simulink model "task_simulation"  (R2025b)
settings: Solver=FixedStepAuto  StartTime=0.0  StopTime=20  FixedStep=Ts * 0.1  RelTol=1e-3
InitFcn:
  | % modelling
  | % design_cascade_control
undefined symbols (not defined in the file): CTRL, I_max_val, J_1_val, J_2_val, k_E_val, k_M_val, k_t_val, L_val, R_val, U_max_val
libraries: slpidlib x7, embmathops x2, simulink_extras x2, simulink x2
settings Model: Creator=10120  LastModifiedBy=10120
settings SolverCC: ZeroCrossAlgorithm=Adaptive
settings DebuggingCC: IgnoredZcDiagnostic=none

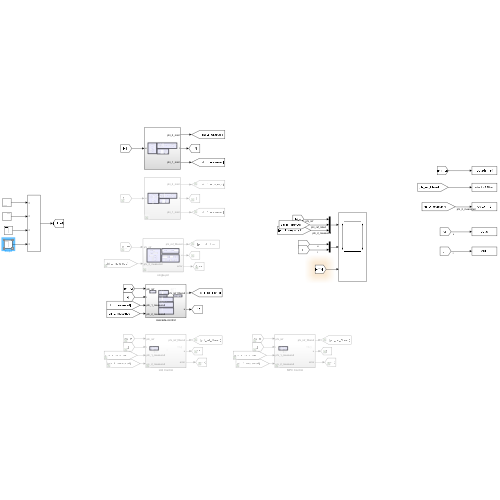
[thumbnail: Simulink's stored preview of the top-level diagram]
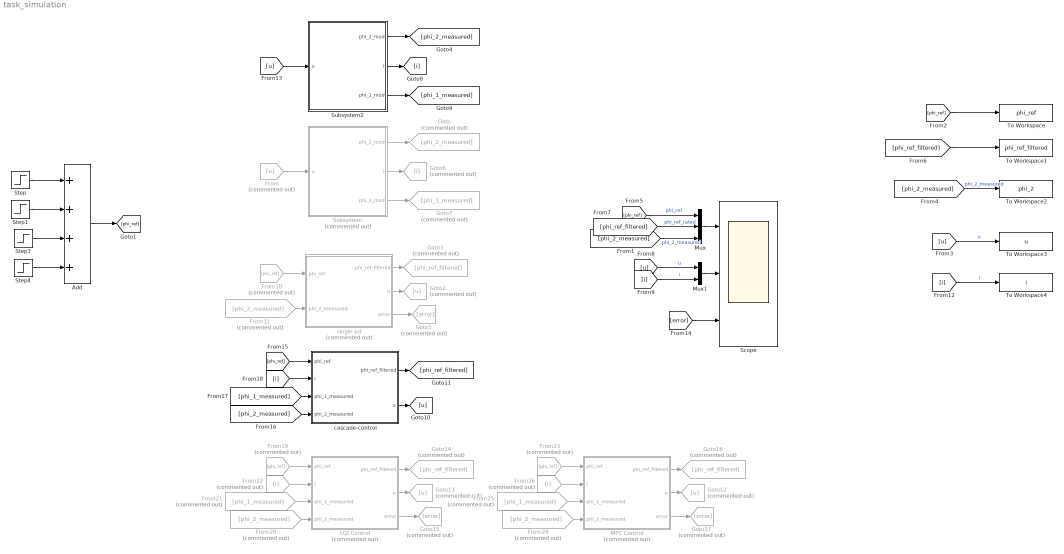
== system task_simulation ==
  Add : Sum  Inputs=++++
  From : From  Commented=on  GotoTag=u
  From10 : From  Commented=on  GotoTag=phi_ref
  From11 : From  Commented=on  GotoTag=phi_2_measured
  From19 : From  Commented=on  GotoTag=phi_ref
  From20 : From  Commented=on  GotoTag=phi_2_measured
  From21 : From  Commented=on  GotoTag=phi_1_measured
  From22 : From  Commented=on  GotoTag=i
  From23 : From  Commented=on  GotoTag=phi_ref
  From24 : From  Commented=on  GotoTag=phi_2_measured
  From25 : From  Commented=on  GotoTag=phi_1_measured
  From26 : From  Commented=on  GotoTag=i
  Goto : Goto  Commented=on  GotoTag=phi_2_measured
  Goto12 : Goto  Commented=on  GotoTag=u
  Goto13 : Goto  Commented=on  GotoTag=u
  Goto14 : Goto  Commented=on  GotoTag=phi_ref_filtered
  Goto15 : Goto  Commented=on  GotoTag=error
  Goto16 : Goto  Commented=on  GotoTag=phi_ref_filtered
  Goto17 : Goto  Commented=on  GotoTag=error
  Goto2 : Goto  Commented=on  GotoTag=u
  Goto3 : Goto  Commented=on  GotoTag=phi_ref_filtered
  Goto5 : Goto  Commented=on  GotoTag=error
  Goto6 : Goto  Commented=on  GotoTag=i
  Goto7 : Goto  Commented=on  GotoTag=phi_1_measured
  LQI Control : Subsystem  Commented=on
  MPC Control : Subsystem  Commented=on
  Mux : Mux  Inputs=3
  Mux1 : Mux  Inputs=2
  Scope : Scope  NumInputPorts=3
      settings: ActiveDisplayYMinimum=-0.74999999999999978  ActiveDisplayYMaximum=6.75
  Step : Step  Time=0.1  After=2  SampleTime=0
  Step1 : Step  Time=5  After=2  SampleTime=0
  Step3 : Step  Time=10  After=-2  SampleTime=0
  Step4 : Step  Time=15  After=-2  SampleTime=0
  Subsystem : Subsystem  Commented=on
  Subsystem2 : Subsystem
  To Workspace : ToWorkspace  VariableName=phi_ref  SaveFormat=Structure With Time  SampleTime=-1
  To Workspace1 : ToWorkspace  VariableName=phi_ref_filtered  SaveFormat=Structure With Time  SampleTime=-1
  To Workspace2 : ToWorkspace  VariableName=phi_2  SaveFormat=Structure With Time  SampleTime=-1
  To Workspace3 : ToWorkspace  VariableName=u  SaveFormat=Structure With Time  SampleTime=-1
  To Workspace4 : ToWorkspace  VariableName=i  SaveFormat=Structure With Time  SampleTime=-1
  cascade-control : Subsystem
  single-pd : Subsystem  Commented=on
  wires:
  From/1 -> Subsystem/1(u)
  Subsystem/1(phi_2_mod) -> Goto/1
  Mux/1 -> Scope/1
  [phi_ref] -> Mux/1  "phi_ref"
  [phi_ref_filtered] -> Mux/2  "phi_ref_rated"
  [phi_2_measured] -> Mux/3  "phi_2_measured"
  Subsystem/2(i) -> Goto6/1
  From10/1 -> single-pd/1(phi_ref)
  From11/1 -> single-pd/2(phi_2_measured)
  single-pd/2(u) -> Goto2/1
  single-pd/1(phi_ref_filtered) -> Goto3/1
  Mux1/1 -> Scope/2
  [u] -> Mux1/1  "u"
  [i] -> Mux1/2  "i"
  [phi_ref] -> To Workspace/1
  [phi_ref_filtered] -> To Workspace1/1
  [phi_2_measured] -> To Workspace2/1  "phi_2_measured"
  [u] -> To Workspace3/1  "u"
  [i] -> To Workspace4/1  "i"
  single-pd/3(error) -> Goto5/1
  [error] -> Scope/3
  Subsystem/3(phi_1_mod) -> Goto7/1
  Subsystem2/3(phi_1_mod) -> [phi_1_measured]
  Subsystem2/2(i) -> [i]
  Subsystem2/1(phi_2_mod) -> [phi_2_measured]
  [u] -> Subsystem2/1(u)
  [phi_ref] -> cascade-control/1(phi_ref)
  cascade-control/1(phi_ref_filtered) -> [phi_ref_filtered]
  [phi_2_measured] -> cascade-control/4(phi_2_measured)
  cascade-control/2(u) -> [u]
  [phi_1_measured] -> cascade-control/3(phi_1_measured)
  [i] -> cascade-control/2(i)
  From22/1 -> LQI Control/2(i)
  LQI Control/1(phi_ref_filtered) -> Goto14/1
  From21/1 -> LQI Control/3(phi_1_measured)
  LQI Control/2(u) -> Goto13/1
  From19/1 -> LQI Control/1(phi_ref)
  From20/1 -> LQI Control/4(phi_2_measured)
  LQI Control/3(error) -> Goto15/1
  From25/1 -> MPC Control/3(phi_1_measured)
  From23/1 -> MPC Control/1(phi_ref)
  MPC Control/1(phi_ref_filtered) -> Goto16/1
  From24/1 -> MPC Control/4(phi_2_measured)
  MPC Control/2(u) -> Goto12/1
  From26/1 -> MPC Control/2(i)
  MPC Control/3(error) -> Goto17/1
  Step/1 -> Add/1
  Step1/1 -> Add/2
  Step3/1 -> Add/3
  Step4/1 -> Add/4
  Add/1 -> [phi_ref]

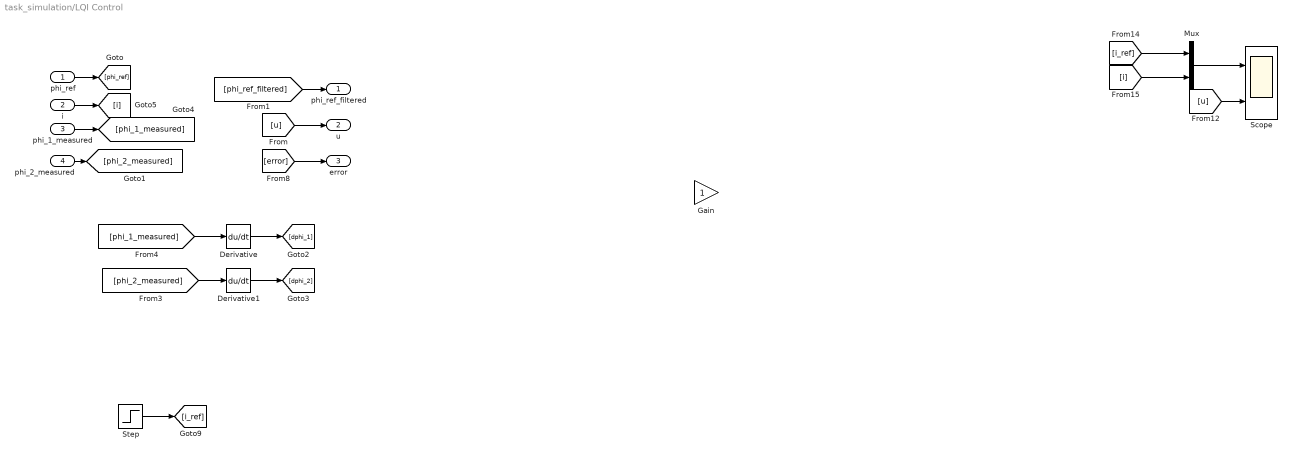
== system task_simulation/LQI Control ==
  phi_ref : Inport
  i : Inport  Port=2
  phi_1_measured : Inport  Port=3
  phi_2_measured : Inport  Port=4
  Derivative : Derivative
  Derivative1 : Derivative
  Gain : Gain
  Mux : Mux  Inputs=2
  Scope : Scope  NumInputPorts=2
      settings: ActiveDisplayYMinimum=-0.12500000000858569  ActiveDisplayYMaximum=1.1250000000772715
  Step : Step  SampleTime=0
  phi_ref_filtered : Outport
  u : Outport  Port=2
  error : Outport  Port=3
  wires:
  phi_ref/1 -> [phi_ref]
  phi_2_measured/1 -> [phi_2_measured]
  [phi_ref_filtered] -> phi_ref_filtered/1
  [u] -> u/1
  [error] -> error/1
  [phi_1_measured] -> Derivative/1
  Derivative/1 -> [dphi_1]
  [phi_2_measured] -> Derivative1/1
  Derivative1/1 -> [dphi_2]
  phi_1_measured/1 -> [phi_1_measured]
  i/1 -> [i]
  [i_ref] -> Mux/1
  [i] -> Mux/2
  Mux/1 -> Scope/1
  [u] -> Scope/2
  Step/1 -> [i_ref]

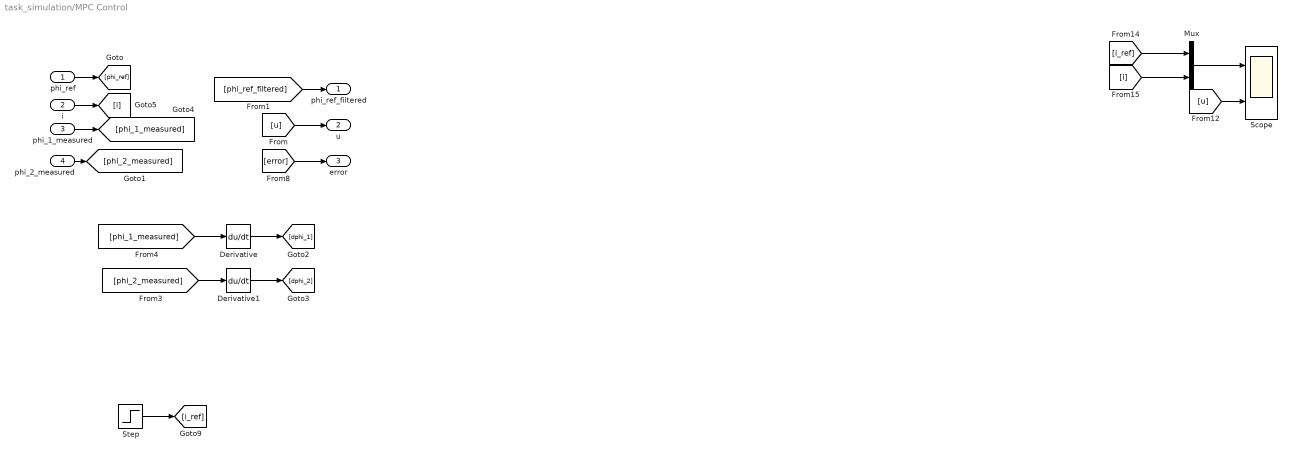
== system task_simulation/MPC Control ==
  phi_ref : Inport
  i : Inport  Port=2
  phi_1_measured : Inport  Port=3
  phi_2_measured : Inport  Port=4
  Derivative : Derivative
  Derivative1 : Derivative
  Mux : Mux  Inputs=2
  Scope : Scope  NumInputPorts=2
      settings: ActiveDisplayYMinimum=-0.12500000000858569  ActiveDisplayYMaximum=1.1250000000772715
  Step : Step  SampleTime=0
  phi_ref_filtered : Outport
  u : Outport  Port=2
  error : Outport  Port=3
  wires:
  phi_ref/1 -> [phi_ref]
  phi_2_measured/1 -> [phi_2_measured]
  [phi_ref_filtered] -> phi_ref_filtered/1
  [u] -> u/1
  [error] -> error/1
  [phi_1_measured] -> Derivative/1
  Derivative/1 -> [dphi_1]
  [phi_2_measured] -> Derivative1/1
  Derivative1/1 -> [dphi_2]
  phi_1_measured/1 -> [phi_1_measured]
  i/1 -> [i]
  [i_ref] -> Mux/1
  [i] -> Mux/2
  Mux/1 -> Scope/1
  [u] -> Scope/2
  Step/1 -> [i_ref]

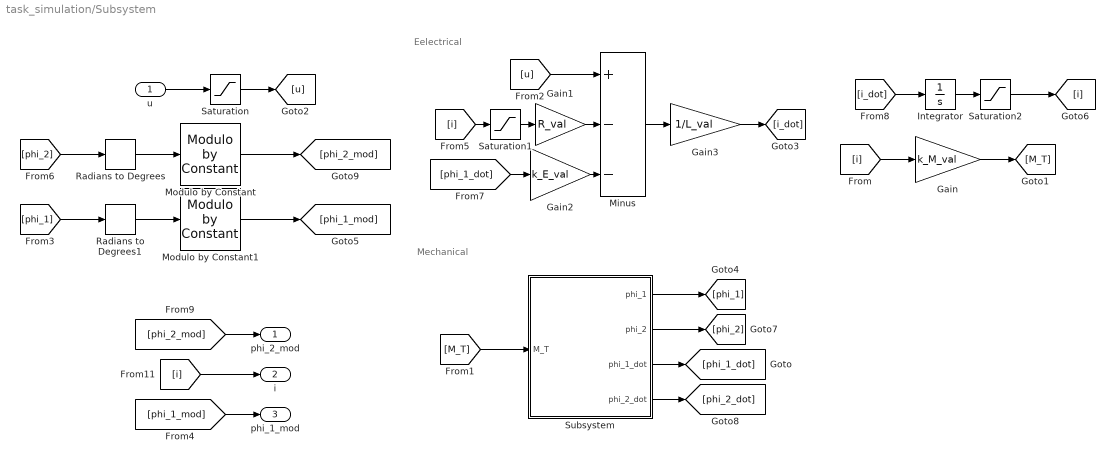
== system task_simulation/Subsystem ==
  note: Mechanical
  note: Eelectrical
  u : Inport
  Gain : Gain  Gain=k_M_val
  Gain1 : Gain  Gain=R_val
  Gain2 : Gain  Gain=k_E_val
  Gain3 : Gain  Gain=1/L_val
  Integrator : Integrator
  Minus : Sum  Inputs=+--
  Modulo by Constant : embmathops/Modulo by Constant  Denominator=360  SimulateUsing=Code generation
      settings: LibrarySourceBlock=embeddedMathLib/Modulo by Constant
  Modulo by Constant1 : embmathops/Modulo by Constant  Denominator=360  SimulateUsing=Code generation
      settings: LibrarySourceBlock=embeddedMathLib/Modulo by Constant
  Radians to Degrees : simulink_extras/Transformations/Radians to Degrees
  Radians to Degrees1 : simulink_extras/Transformations/Radians to Degrees
  Saturation : Saturate  UpperLimit=U_max_val  LowerLimit=-U_max_val
  Saturation1 : Saturate  UpperLimit=I_max_val  LowerLimit=-I_max_val
  Saturation2 : Saturate  UpperLimit=I_max_val  LowerLimit=-I_max_val
  Subsystem : Subsystem
  phi_2_mod : Outport
  i : Outport  Port=2
  phi_1_mod : Outport  Port=3
  wires:
  [i] -> Gain/1
  Gain/1 -> [M_T]
  [M_T] -> Subsystem/1(M_T)
  u/1 -> Saturation/1
  Gain3/1 -> [i_dot]
  [u] -> Minus/1
  Gain1/1 -> Minus/2
  [i] -> Saturation1/1
  Subsystem/1(phi_1) -> [phi_1]
  Gain2/1 -> Minus/3
  [phi_1_dot] -> Gain2/1
  Minus/1 -> Gain3/1
  [i_dot] -> Integrator/1
  Integrator/1 -> Saturation2/1
  Subsystem/3(phi_1_dot) -> [phi_1_dot]
  [phi_2_mod] -> phi_2_mod/1
  Subsystem/2(phi_2) -> [phi_2]
  Subsystem/4(phi_2_dot) -> [phi_2_dot]
  [phi_2] -> Radians to Degrees/1
  Saturation/1 -> [u]
  Saturation1/1 -> Gain1/1
  Saturation2/1 -> [i]
  [i] -> i/1
  Radians to Degrees/1 -> Modulo by Constant/1
  Modulo by Constant/1 -> [phi_2_mod]
  Radians to Degrees1/1 -> Modulo by Constant1/1
  [phi_1] -> Radians to Degrees1/1
  Modulo by Constant1/1 -> [phi_1_mod]
  [phi_1_mod] -> phi_1_mod/1

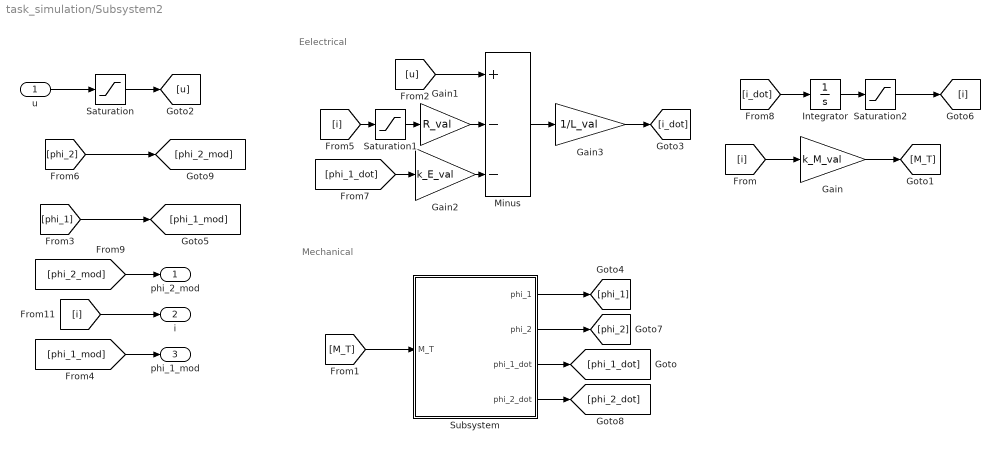
== system task_simulation/Subsystem2 ==
  note: Mechanical
  note: Eelectrical
  u : Inport
  Gain : Gain  Gain=k_M_val
  Gain1 : Gain  Gain=R_val
  Gain2 : Gain  Gain=k_E_val
  Gain3 : Gain  Gain=1/L_val
  Integrator : Integrator
  Minus : Sum  Inputs=+--
  Saturation : Saturate  UpperLimit=U_max_val  LowerLimit=-U_max_val
  Saturation1 : Saturate  UpperLimit=I_max_val  LowerLimit=-I_max_val
  Saturation2 : Saturate  UpperLimit=I_max_val  LowerLimit=-I_max_val
  Subsystem : Subsystem
  phi_2_mod : Outport
  i : Outport  Port=2
  phi_1_mod : Outport  Port=3
  wires:
  [i] -> Gain/1
  Gain/1 -> [M_T]
  [M_T] -> Subsystem/1(M_T)
  u/1 -> Saturation/1
  Gain3/1 -> [i_dot]
  [u] -> Minus/1
  Gain1/1 -> Minus/2
  [i] -> Saturation1/1
  Subsystem/1(phi_1) -> [phi_1]
  Gain2/1 -> Minus/3
  [phi_1_dot] -> Gain2/1
  Minus/1 -> Gain3/1
  [i_dot] -> Integrator/1
  Integrator/1 -> Saturation2/1
  Subsystem/3(phi_1_dot) -> [phi_1_dot]
  [phi_2_mod] -> phi_2_mod/1
  Subsystem/2(phi_2) -> [phi_2]
  Subsystem/4(phi_2_dot) -> [phi_2_dot]
  Saturation/1 -> [u]
  Saturation1/1 -> Gain1/1
  Saturation2/1 -> [i]
  [i] -> i/1
  [phi_2] -> [phi_2_mod]
  [phi_1] -> [phi_1_mod]
  [phi_1_mod] -> phi_1_mod/1

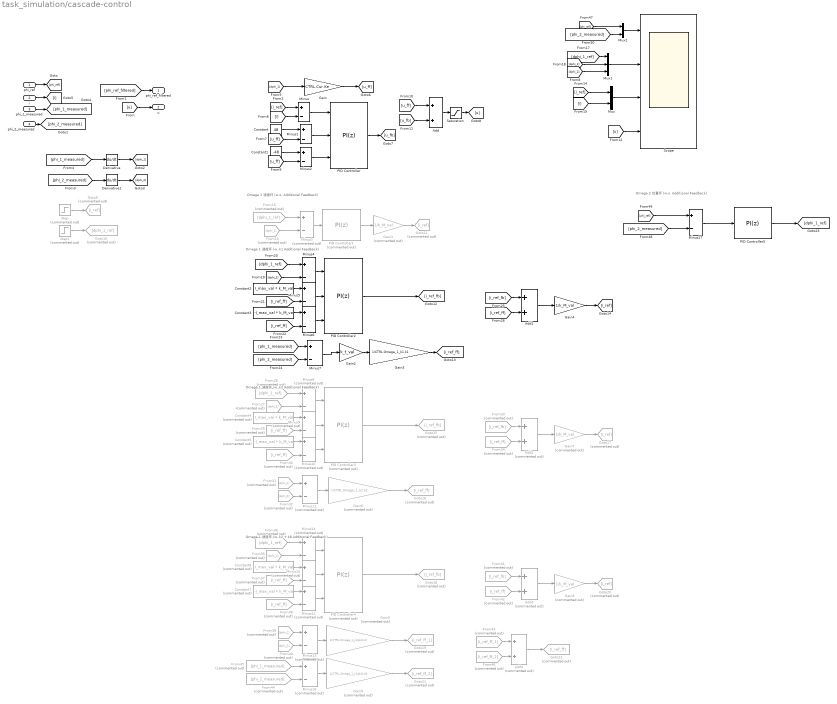
== system task_simulation/cascade-control ==
  note: Omega 1 速度环 (w. k1 Additional Feedback)
  note: Omega 1 速度环 (w.o. Additional Feedback)
  note: Omega 1 速度环 (w. k2 Additional Feedback)
  note: Omega 1 速度环 (w. k2 + k8 Additional Feedback)
  note: Omega 2 位置环 (w.o. Additional Feedback)
  phi_ref : Inport
  i : Inport  Port=2
  phi_1_measured : Inport  Port=3
  phi_2_measured : Inport  Port=4
  Add : Sum
  Add1 : Sum
  Add2 : Sum  Commented=on
  Add3 : Sum  Commented=on
  Add4 : Sum  Commented=on
  Constant : Constant  Value=48
  Constant1 : Constant  Value=-48
  Constant2 : Constant  Value=I_max_val * k_M_val
  Constant3 : Constant  Value=-I_max_val * k_M_val
  Constant4 : Constant  Commented=on  Value=I_max_val * k_M_val
  Constant5 : Constant  Commented=on  Value=-I_max_val * k_M_val
  Constant6 : Constant  Commented=on  Value=I_max_val * k_M_val
  Constant7 : Constant  Commented=on  Value=-I_max_val * k_M_val
  Derivative : Derivative
  Derivative1 : Derivative
  From{13,27,31,35,39} (5 alike) : From  Commented=on  GotoTag=dphi_1
  From16 : From  Commented=on  GotoTag=dphi_1_ref
  From28 : From  Commented=on  GotoTag=dphi_1_ref
  From{29..30,34,37..38,42} (6 alike) : From  Commented=on  GotoTag=i_ref_ff
  From32 : From  Commented=on  GotoTag=dphi_2
  From33 : From  Commented=on  GotoTag=i_ref_fb
  From36 : From  Commented=on  GotoTag=dphi_1_ref
  From40 : From  Commented=on  GotoTag=dphi_2
  From41 : From  Commented=on  GotoTag=i_ref_fb
  From43 : From  Commented=on  GotoTag=i_ref_ff_1
  From44 : From  Commented=on  GotoTag=phi_2_measured
  From45 : From  Commented=on  GotoTag=phi_1_measured
  From46 : From  Commented=on  GotoTag=i_ref_ff_2
  Gain : Gain  Gain=CTRL.Cur.Ke
  Gain1 : Gain  Commented=on  Gain=1/k_M_val
  Gain2 : Gain  Gain=k_t_val
  Gain3 : Gain  Gain=1/CTRL.Omega_1_k1.k1
  Gain4 : Gain  Gain=1/k_M_val
  Gain5 : Gain  Commented=on  Gain=1/CTRL.Omega_1_k2pk8.k2
  Gain6 : Gain  Commented=on  Gain=1/CTRL.Omega_1_k2.k2
  Gain7 : Gain  Commented=on  Gain=1/k_M_val
  Gain8 : Gain  Commented=on  Gain=1/k_M_val
  Gain9 : Gain  Commented=on  Gain=1/CTRL.Omega_1_k2pk8.k8
  Goto10 : Goto  Commented=on  GotoTag=dphi_1_ref
  Goto{9,11,17,20} (4 alike) : Goto  Commented=on  GotoTag=i_ref
  Goto15 : Goto  Commented=on  GotoTag=i_ref_fb
  Goto16 : Goto  Commented=on  GotoTag=i_ref_ff
  Goto18 : Goto  Commented=on  GotoTag=i_ref_fb
  Goto19 : Goto  Commented=on  GotoTag=i_ref_ff_1
  Goto21 : Goto  Commented=on  GotoTag=i_ref_ff_2
  Goto22 : Goto  Commented=on  GotoTag=i_ref_ff
  Minus{,1..2,4..7,17} (8 alike) : Sum  Inputs=+-
  Minus{3,8..16} (10 alike) : Sum  Commented=on  Inputs=+-
  Mux : Mux  Inputs=2
  Mux1 : Mux  Inputs=3
  Mux2 : Mux  Inputs=2
  PID Controller : slpidlib/PID Controller  Controller=PI  Form=Parallel  TimeDomain=Discrete-time  UseExternalTs=off  SampleTime=-1  IntegratorMethod=Forward Euler  FilterMethod=Forward Euler  ControllerParametersSource=internal  P=CTRL.Cur.Kp  I=CTRL.Cur.Ki  UseKiTs=off  D=0  UseExternalDerivativeSource=off  N=100  UseFilter=on  TunerSelectOption=Transfer Function Based (PID Tuner App)  InitialConditionSource=internal  InitialConditionForIntegrator=0  InitialConditionForFilter=0  DifferentiatorICPrevScaledInput=0  ExternalReset=none  TrackingMode=off  Kt=1  LimitOutput=on  SatLimitsSource=external  UpperSaturationLimit=inf  LowerSaturationLimit=-inf  LinearizeAsGain=on  AntiWindupMode=clamping  Kb=1  LimitIntegrator=off  UpperIntegratorSaturationLimit=inf  LowerIntegratorSaturationLimit=-inf  POutMin=[]  POutMax=[]  IOutMin=[]  IOutMax=[]  DOutMin=[]  DOutMax=[]  NOutMin=[]  NOutMax=[]  SumOutMin=[]  SumOutMax=[]  SaturationOutMin=[]  SaturationOutMax=[]  PParamMin=[]  PParamMax=[]  IParamMin=[]  IParamMax=[]  DParamMin=[]  DParamMax=[]  NParamMin=[]  NParamMax=[]  KbParamMin=[]  KbParamMax=[]  KtParamMin=[]  KtParamMax=[]  KbOutMin=[]  KbOutMax=[]  KtOutMin=[]  KtOutMax=[]  IntegratorOutMin=[]  IntegratorOutMax=[]  FilterOutMin=[]  FilterOutMax=[]  SumI1OutMin=[]  SumI1OutMax=[]  SumI2OutMin=[]  SumI2OutMax=[]  SumI3OutMin=[]  SumI3OutMax=[]  SumI4OutMin=[]  SumI4OutMax=[]  SumDOutMin=[]  SumDOutMax=[]  DifferentiatorOutMin=[]  DifferentiatorOutMax=[]  FilterDiffOutCoefMin=[]  FilterDiffOutCoefMax=[]  ReciprocalOutMin=[]  ReciprocalOutMax=[]  SumDenOutMin=[]  SumDenOutMax=[]  SumNumOutMin=[]  SumNumOutMax=[]  DivideOutMin=[]  DivideOutMax=[]  UdiffTsProdOutMin=[]  UdiffTsProdOutMax=[]  NTsProdOutMin=[]  NTsProdOutMax=[]  UintegralTsProdOutMin=[]  UintegralTsProdOutMax=[]  UngainTsProdOutMin=[]  UngainTsProdOutMax=[]  ClampingZeroOutDataTypeStr=Inherit: Inherit via back propagation  ClampingZeroOutMin=[]  ClampingZeroOutMax=[]  FilterDenConstantOutDataTypeStr=Inherit: Inherit via back propagation  FilterDenConstantOutMin=[]  FilterDenConstantOutMax=[]  PCopyOutDataTypeStr=Inherit: Inherit via back propagation  PCopyOutMin=[]  PCopyOutMax=[]  NCopyOutDataTypeStr=Inherit: Inherit via back propagation  NCopyOutMin=[]  NCopyOutMax=[]  IntegratorContinuousStateAttributes=''  IntegratorStateMustResolveToSignalObject=off  IntegratorRTWStateStorageClass=Auto  FilterContinuousStateAttributes=''  FilterStateMustResolveToSignalObject=off  FilterRTWStateStorageClass=Auto  ParallelPVariant=InternalParameters  IdealPVariant=Disabled  IVariant=InternalParameters  DVariant=Disabled  IntegratorVariant=Discrete  SatVariant=External  AWVariant=DiscClampingParallel  PCopyVariant=Disabled  TRVariant=Disabled  FdbkBlocksVariant=Forward  IdealPFdbkVariant=Disabled  SatFdbkVariant=Disabled  DerivativeFilterVariant=Disabled  NVariant=Disabled  NCopyVariant=Disabled_SignalSpec  FilterICVariant=Disabled  IntegratorICVariant=InternalICs  ExternalResetVariant=Disabled  TRSumVariant=Passthrough  SumFdbkVariant=Disabled  SumVariant=Sum_PI  TsampFilterVariant=InternalTs  TsampNgainVariant=Passthrough  TsampIntegralVariant=Disabled_SignalSpec  ExternalSaturationOutDataTypeStr=Inherit: Same as second input  DerivativeSourceVariant=Disabled  PreIntVariant=InternalPreInt
  PID Controller1 : slpidlib/PID Controller  Commented=on  Controller=PI  Form=Parallel  TimeDomain=Discrete-time  UseExternalTs=off  SampleTime=-1  IntegratorMethod=Forward Euler  FilterMethod=Forward Euler  ControllerParametersSource=internal  P=CTRL.Omega_1.Kp  I=CTRL.Omega_1.Ki  UseKiTs=off  D=0  UseExternalDerivativeSource=off  N=100  UseFilter=on  TunerSelectOption=Transfer Function Based (PID Tuner App)  InitialConditionSource=internal  InitialConditionForIntegrator=0  InitialConditionForFilter=0  DifferentiatorICPrevScaledInput=0  ExternalReset=none  TrackingMode=off  Kt=1  LimitOutput=on  SatLimitsSource=internal  UpperSaturationLimit=I_max_val * k_M_val  LowerSaturationLimit=-I_max_val * k_M_val  LinearizeAsGain=on  AntiWindupMode=clamping  Kb=1  LimitIntegrator=off  UpperIntegratorSaturationLimit=inf  LowerIntegratorSaturationLimit=-inf  POutMin=[]  POutMax=[]  IOutMin=[]  IOutMax=[]  DOutMin=[]  DOutMax=[]  NOutMin=[]  NOutMax=[]  SumOutMin=[]  SumOutMax=[]  SaturationOutMin=[]  SaturationOutMax=[]  PParamMin=[]  PParamMax=[]  IParamMin=[]  IParamMax=[]  DParamMin=[]  DParamMax=[]  NParamMin=[]  NParamMax=[]  KbParamMin=[]  KbParamMax=[]  KtParamMin=[]  KtParamMax=[]  KbOutMin=[]  KbOutMax=[]  KtOutMin=[]  KtOutMax=[]  IntegratorOutMin=[]  IntegratorOutMax=[]  FilterOutMin=[]  FilterOutMax=[]  SumI1OutMin=[]  SumI1OutMax=[]  SumI2OutMin=[]  SumI2OutMax=[]  SumI3OutMin=[]  SumI3OutMax=[]  SumI4OutMin=[]  SumI4OutMax=[]  SumDOutMin=[]  SumDOutMax=[]  DifferentiatorOutMin=[]  DifferentiatorOutMax=[]  FilterDiffOutCoefMin=[]  FilterDiffOutCoefMax=[]  ReciprocalOutMin=[]  ReciprocalOutMax=[]  SumDenOutMin=[]  SumDenOutMax=[]  SumNumOutMin=[]  SumNumOutMax=[]  DivideOutMin=[]  DivideOutMax=[]  UdiffTsProdOutMin=[]  UdiffTsProdOutMax=[]  NTsProdOutMin=[]  NTsProdOutMax=[]  UintegralTsProdOutMin=[]  UintegralTsProdOutMax=[]  UngainTsProdOutMin=[]  UngainTsProdOutMax=[]  ClampingZeroOutDataTypeStr=Inherit: Inherit via back propagation  ClampingZeroOutMin=[]  ClampingZeroOutMax=[]  FilterDenConstantOutDataTypeStr=Inherit: Inherit via back propagation  FilterDenConstantOutMin=[]  FilterDenConstantOutMax=[]  PCopyOutDataTypeStr=Inherit: Inherit via back propagation  PCopyOutMin=[]  PCopyOutMax=[]  NCopyOutDataTypeStr=Inherit: Inherit via back propagation  NCopyOutMin=[]  NCopyOutMax=[]  IntegratorContinuousStateAttributes=''  IntegratorStateMustResolveToSignalObject=off  IntegratorRTWStateStorageClass=Auto  FilterContinuousStateAttributes=''  FilterStateMustResolveToSignalObject=off  FilterRTWStateStorageClass=Auto  ParallelPVariant=InternalParameters  IdealPVariant=Disabled  IVariant=InternalParameters  DVariant=Disabled  IntegratorVariant=Discrete  SatVariant=Enabled  AWVariant=DiscClampingParallel  PCopyVariant=Disabled  TRVariant=Disabled  FdbkBlocksVariant=Forward  IdealPFdbkVariant=Disabled  SatFdbkVariant=Disabled  DerivativeFilterVariant=Disabled  NVariant=Disabled  NCopyVariant=Disabled_SignalSpec  FilterICVariant=Disabled  IntegratorICVariant=InternalICs  ExternalResetVariant=Disabled  TRSumVariant=Passthrough  SumFdbkVariant=Disabled  SumVariant=Sum_PI  TsampFilterVariant=InternalTs  TsampNgainVariant=Passthrough  TsampIntegralVariant=Disabled_SignalSpec  ExternalSaturationOutDataTypeStr=Inherit: Same as second input  DerivativeSourceVariant=Disabled  PreIntVariant=InternalPreInt
  PID Controller2 : slpidlib/PID Controller  Controller=PI  Form=Parallel  TimeDomain=Discrete-time  UseExternalTs=off  SampleTime=-1  IntegratorMethod=Forward Euler  FilterMethod=Forward Euler  ControllerParametersSource=internal  P=CTRL.Omega_1_k1.Kp  I=CTRL.Omega_1_k1.Ki  UseKiTs=off  D=0  UseExternalDerivativeSource=off  N=100  UseFilter=on  TunerSelectOption=Transfer Function Based (PID Tuner App)  InitialConditionSource=internal  InitialConditionForIntegrator=0  InitialConditionForFilter=0  DifferentiatorICPrevScaledInput=0  ExternalReset=none  TrackingMode=off  Kt=1  LimitOutput=on  SatLimitsSource=external  UpperSaturationLimit=I_max_val * k_M_val  LowerSaturationLimit=-I_max_val * k_M_val  LinearizeAsGain=on  AntiWindupMode=clamping  Kb=1  LimitIntegrator=off  UpperIntegratorSaturationLimit=inf  LowerIntegratorSaturationLimit=-inf  POutMin=[]  POutMax=[]  IOutMin=[]  IOutMax=[]  DOutMin=[]  DOutMax=[]  NOutMin=[]  NOutMax=[]  SumOutMin=[]  SumOutMax=[]  SaturationOutMin=[]  SaturationOutMax=[]  PParamMin=[]  PParamMax=[]  IParamMin=[]  IParamMax=[]  DParamMin=[]  DParamMax=[]  NParamMin=[]  NParamMax=[]  KbParamMin=[]  KbParamMax=[]  KtParamMin=[]  KtParamMax=[]  KbOutMin=[]  KbOutMax=[]  KtOutMin=[]  KtOutMax=[]  IntegratorOutMin=[]  IntegratorOutMax=[]  FilterOutMin=[]  FilterOutMax=[]  SumI1OutMin=[]  SumI1OutMax=[]  SumI2OutMin=[]  SumI2OutMax=[]  SumI3OutMin=[]  SumI3OutMax=[]  SumI4OutMin=[]  SumI4OutMax=[]  SumDOutMin=[]  SumDOutMax=[]  DifferentiatorOutMin=[]  DifferentiatorOutMax=[]  FilterDiffOutCoefMin=[]  FilterDiffOutCoefMax=[]  ReciprocalOutMin=[]  ReciprocalOutMax=[]  SumDenOutMin=[]  SumDenOutMax=[]  SumNumOutMin=[]  SumNumOutMax=[]  DivideOutMin=[]  DivideOutMax=[]  UdiffTsProdOutMin=[]  UdiffTsProdOutMax=[]  NTsProdOutMin=[]  NTsProdOutMax=[]  UintegralTsProdOutMin=[]  UintegralTsProdOutMax=[]  UngainTsProdOutMin=[]  UngainTsProdOutMax=[]  ClampingZeroOutDataTypeStr=Inherit: Inherit via back propagation  ClampingZeroOutMin=[]  ClampingZeroOutMax=[]  FilterDenConstantOutDataTypeStr=Inherit: Inherit via back propagation  FilterDenConstantOutMin=[]  FilterDenConstantOutMax=[]  PCopyOutDataTypeStr=Inherit: Inherit via back propagation  PCopyOutMin=[]  PCopyOutMax=[]  NCopyOutDataTypeStr=Inherit: Inherit via back propagation  NCopyOutMin=[]  NCopyOutMax=[]  IntegratorContinuousStateAttributes=''  IntegratorStateMustResolveToSignalObject=off  IntegratorRTWStateStorageClass=Auto  FilterContinuousStateAttributes=''  FilterStateMustResolveToSignalObject=off  FilterRTWStateStorageClass=Auto  ParallelPVariant=InternalParameters  IdealPVariant=Disabled  IVariant=InternalParameters  DVariant=Disabled  IntegratorVariant=Discrete  SatVariant=External  AWVariant=DiscClampingParallel  PCopyVariant=Disabled  TRVariant=Disabled  FdbkBlocksVariant=Forward  IdealPFdbkVariant=Disabled  SatFdbkVariant=Disabled  DerivativeFilterVariant=Disabled  NVariant=Disabled  NCopyVariant=Disabled_SignalSpec  FilterICVariant=Disabled  IntegratorICVariant=InternalICs  ExternalResetVariant=Disabled  TRSumVariant=Passthrough  SumFdbkVariant=Disabled  SumVariant=Sum_PI  TsampFilterVariant=InternalTs  TsampNgainVariant=Passthrough  TsampIntegralVariant=Disabled_SignalSpec  ExternalSaturationOutDataTypeStr=Inherit: Same as second input  DerivativeSourceVariant=Disabled  PreIntVariant=InternalPreInt
  PID Controller3 : slpidlib/PID Controller  Commented=on  Controller=PI  Form=Parallel  TimeDomain=Discrete-time  UseExternalTs=off  SampleTime=-1  IntegratorMethod=Forward Euler  FilterMethod=Forward Euler  ControllerParametersSource=internal  P=CTRL.Omega_1_k2.Kp  I=CTRL.Omega_1_k2.Ki  UseKiTs=off  D=0  UseExternalDerivativeSource=off  N=100  UseFilter=on  TunerSelectOption=Transfer Function Based (PID Tuner App)  InitialConditionSource=internal  InitialConditionForIntegrator=0  InitialConditionForFilter=0  DifferentiatorICPrevScaledInput=0  ExternalReset=none  TrackingMode=off  Kt=1  LimitOutput=on  SatLimitsSource=external  UpperSaturationLimit=I_max_val * k_M_val  LowerSaturationLimit=-I_max_val * k_M_val  LinearizeAsGain=on  AntiWindupMode=clamping  Kb=1  LimitIntegrator=off  UpperIntegratorSaturationLimit=inf  LowerIntegratorSaturationLimit=-inf  POutMin=[]  POutMax=[]  IOutMin=[]  IOutMax=[]  DOutMin=[]  DOutMax=[]  NOutMin=[]  NOutMax=[]  SumOutMin=[]  SumOutMax=[]  SaturationOutMin=[]  SaturationOutMax=[]  PParamMin=[]  PParamMax=[]  IParamMin=[]  IParamMax=[]  DParamMin=[]  DParamMax=[]  NParamMin=[]  NParamMax=[]  KbParamMin=[]  KbParamMax=[]  KtParamMin=[]  KtParamMax=[]  KbOutMin=[]  KbOutMax=[]  KtOutMin=[]  KtOutMax=[]  IntegratorOutMin=[]  IntegratorOutMax=[]  FilterOutMin=[]  FilterOutMax=[]  SumI1OutMin=[]  SumI1OutMax=[]  SumI2OutMin=[]  SumI2OutMax=[]  SumI3OutMin=[]  SumI3OutMax=[]  SumI4OutMin=[]  SumI4OutMax=[]  SumDOutMin=[]  SumDOutMax=[]  DifferentiatorOutMin=[]  DifferentiatorOutMax=[]  FilterDiffOutCoefMin=[]  FilterDiffOutCoefMax=[]  ReciprocalOutMin=[]  ReciprocalOutMax=[]  SumDenOutMin=[]  SumDenOutMax=[]  SumNumOutMin=[]  SumNumOutMax=[]  DivideOutMin=[]  DivideOutMax=[]  UdiffTsProdOutMin=[]  UdiffTsProdOutMax=[]  NTsProdOutMin=[]  NTsProdOutMax=[]  UintegralTsProdOutMin=[]  UintegralTsProdOutMax=[]  UngainTsProdOutMin=[]  UngainTsProdOutMax=[]  ClampingZeroOutDataTypeStr=Inherit: Inherit via back propagation  ClampingZeroOutMin=[]  ClampingZeroOutMax=[]  FilterDenConstantOutDataTypeStr=Inherit: Inherit via back propagation  FilterDenConstantOutMin=[]  FilterDenConstantOutMax=[]  PCopyOutDataTypeStr=Inherit: Inherit via back propagation  PCopyOutMin=[]  PCopyOutMax=[]  NCopyOutDataTypeStr=Inherit: Inherit via back propagation  NCopyOutMin=[]  NCopyOutMax=[]  IntegratorContinuousStateAttributes=''  IntegratorStateMustResolveToSignalObject=off  IntegratorRTWStateStorageClass=Auto  FilterContinuousStateAttributes=''  FilterStateMustResolveToSignalObject=off  FilterRTWStateStorageClass=Auto  ParallelPVariant=InternalParameters  IdealPVariant=Disabled  IVariant=InternalParameters  DVariant=Disabled  IntegratorVariant=Discrete  SatVariant=External  AWVariant=DiscClampingParallel  PCopyVariant=Disabled  TRVariant=Disabled  FdbkBlocksVariant=Forward  IdealPFdbkVariant=Disabled  SatFdbkVariant=Disabled  DerivativeFilterVariant=Disabled  NVariant=Disabled  NCopyVariant=Disabled_SignalSpec  FilterICVariant=Disabled  IntegratorICVariant=InternalICs  ExternalResetVariant=Disabled  TRSumVariant=Passthrough  SumFdbkVariant=Disabled  SumVariant=Sum_PI  TsampFilterVariant=InternalTs  TsampNgainVariant=Passthrough  TsampIntegralVariant=Disabled_SignalSpec  ExternalSaturationOutDataTypeStr=Inherit: Same as second input  DerivativeSourceVariant=Disabled  PreIntVariant=InternalPreInt
  PID Controller4 : slpidlib/PID Controller  Commented=on  Controller=PI  Form=Parallel  TimeDomain=Discrete-time  UseExternalTs=off  SampleTime=-1  IntegratorMethod=Forward Euler  FilterMethod=Forward Euler  ControllerParametersSource=internal  P=CTRL.Omega_1_k2pk8.Kp  I=CTRL.Omega_1_k2pk8.Ki  UseKiTs=off  D=0  UseExternalDerivativeSource=off  N=100  UseFilter=on  TunerSelectOption=Transfer Function Based (PID Tuner App)  InitialConditionSource=internal  InitialConditionForIntegrator=0  InitialConditionForFilter=0  DifferentiatorICPrevScaledInput=0  ExternalReset=none  TrackingMode=off  Kt=1  LimitOutput=on  SatLimitsSource=external  UpperSaturationLimit=I_max_val * k_M_val  LowerSaturationLimit=-I_max_val * k_M_val  LinearizeAsGain=on  AntiWindupMode=clamping  Kb=1  LimitIntegrator=off  UpperIntegratorSaturationLimit=inf  LowerIntegratorSaturationLimit=-inf  POutMin=[]  POutMax=[]  IOutMin=[]  IOutMax=[]  DOutMin=[]  DOutMax=[]  NOutMin=[]  NOutMax=[]  SumOutMin=[]  SumOutMax=[]  SaturationOutMin=[]  SaturationOutMax=[]  PParamMin=[]  PParamMax=[]  IParamMin=[]  IParamMax=[]  DParamMin=[]  DParamMax=[]  NParamMin=[]  NParamMax=[]  KbParamMin=[]  KbParamMax=[]  KtParamMin=[]  KtParamMax=[]  KbOutMin=[]  KbOutMax=[]  KtOutMin=[]  KtOutMax=[]  IntegratorOutMin=[]  IntegratorOutMax=[]  FilterOutMin=[]  FilterOutMax=[]  SumI1OutMin=[]  SumI1OutMax=[]  SumI2OutMin=[]  SumI2OutMax=[]  SumI3OutMin=[]  SumI3OutMax=[]  SumI4OutMin=[]  SumI4OutMax=[]  SumDOutMin=[]  SumDOutMax=[]  DifferentiatorOutMin=[]  DifferentiatorOutMax=[]  FilterDiffOutCoefMin=[]  FilterDiffOutCoefMax=[]  ReciprocalOutMin=[]  ReciprocalOutMax=[]  SumDenOutMin=[]  SumDenOutMax=[]  SumNumOutMin=[]  SumNumOutMax=[]  DivideOutMin=[]  DivideOutMax=[]  UdiffTsProdOutMin=[]  UdiffTsProdOutMax=[]  NTsProdOutMin=[]  NTsProdOutMax=[]  UintegralTsProdOutMin=[]  UintegralTsProdOutMax=[]  UngainTsProdOutMin=[]  UngainTsProdOutMax=[]  ClampingZeroOutDataTypeStr=Inherit: Inherit via back propagation  ClampingZeroOutMin=[]  ClampingZeroOutMax=[]  FilterDenConstantOutDataTypeStr=Inherit: Inherit via back propagation  FilterDenConstantOutMin=[]  FilterDenConstantOutMax=[]  PCopyOutDataTypeStr=Inherit: Inherit via back propagation  PCopyOutMin=[]  PCopyOutMax=[]  NCopyOutDataTypeStr=Inherit: Inherit via back propagation  NCopyOutMin=[]  NCopyOutMax=[]  IntegratorContinuousStateAttributes=''  IntegratorStateMustResolveToSignalObject=off  IntegratorRTWStateStorageClass=Auto  FilterContinuousStateAttributes=''  FilterStateMustResolveToSignalObject=off  FilterRTWStateStorageClass=Auto  ParallelPVariant=InternalParameters  IdealPVariant=Disabled  IVariant=InternalParameters  DVariant=Disabled  IntegratorVariant=Discrete  SatVariant=External  AWVariant=DiscClampingParallel  PCopyVariant=Disabled  TRVariant=Disabled  FdbkBlocksVariant=Forward  IdealPFdbkVariant=Disabled  SatFdbkVariant=Disabled  DerivativeFilterVariant=Disabled  NVariant=Disabled  NCopyVariant=Disabled_SignalSpec  FilterICVariant=Disabled  IntegratorICVariant=InternalICs  ExternalResetVariant=Disabled  TRSumVariant=Passthrough  SumFdbkVariant=Disabled  SumVariant=Sum_PI  TsampFilterVariant=InternalTs  TsampNgainVariant=Passthrough  TsampIntegralVariant=Disabled_SignalSpec  ExternalSaturationOutDataTypeStr=Inherit: Same as second input  DerivativeSourceVariant=Disabled  PreIntVariant=InternalPreInt
  PID Controller5 : slpidlib/PID Controller  Controller=PI  Form=Parallel  TimeDomain=Discrete-time  UseExternalTs=off  SampleTime=-1  IntegratorMethod=Forward Euler  FilterMethod=Forward Euler  ControllerParametersSource=internal  P=1  I=0  UseKiTs=off  D=0  UseExternalDerivativeSource=off  N=100  UseFilter=on  TunerSelectOption=Transfer Function Based (PID Tuner App)  InitialConditionSource=internal  InitialConditionForIntegrator=0  InitialConditionForFilter=0  DifferentiatorICPrevScaledInput=0  ExternalReset=none  TrackingMode=off  Kt=1  LimitOutput=on  SatLimitsSource=internal  UpperSaturationLimit=I_max_val * k_M_val  LowerSaturationLimit=-I_max_val * k_M_val  LinearizeAsGain=on  AntiWindupMode=clamping  Kb=1  LimitIntegrator=off  UpperIntegratorSaturationLimit=inf  LowerIntegratorSaturationLimit=-inf  POutMin=[]  POutMax=[]  IOutMin=[]  IOutMax=[]  DOutMin=[]  DOutMax=[]  NOutMin=[]  NOutMax=[]  SumOutMin=[]  SumOutMax=[]  SaturationOutMin=[]  SaturationOutMax=[]  PParamMin=[]  PParamMax=[]  IParamMin=[]  IParamMax=[]  DParamMin=[]  DParamMax=[]  NParamMin=[]  NParamMax=[]  KbParamMin=[]  KbParamMax=[]  KtParamMin=[]  KtParamMax=[]  KbOutMin=[]  KbOutMax=[]  KtOutMin=[]  KtOutMax=[]  IntegratorOutMin=[]  IntegratorOutMax=[]  FilterOutMin=[]  FilterOutMax=[]  SumI1OutMin=[]  SumI1OutMax=[]  SumI2OutMin=[]  SumI2OutMax=[]  SumI3OutMin=[]  SumI3OutMax=[]  SumI4OutMin=[]  SumI4OutMax=[]  SumDOutMin=[]  SumDOutMax=[]  DifferentiatorOutMin=[]  DifferentiatorOutMax=[]  FilterDiffOutCoefMin=[]  FilterDiffOutCoefMax=[]  ReciprocalOutMin=[]  ReciprocalOutMax=[]  SumDenOutMin=[]  SumDenOutMax=[]  SumNumOutMin=[]  SumNumOutMax=[]  DivideOutMin=[]  DivideOutMax=[]  UdiffTsProdOutMin=[]  UdiffTsProdOutMax=[]  NTsProdOutMin=[]  NTsProdOutMax=[]  UintegralTsProdOutMin=[]  UintegralTsProdOutMax=[]  UngainTsProdOutMin=[]  UngainTsProdOutMax=[]  ClampingZeroOutDataTypeStr=Inherit: Inherit via back propagation  ClampingZeroOutMin=[]  ClampingZeroOutMax=[]  FilterDenConstantOutDataTypeStr=Inherit: Inherit via back propagation  FilterDenConstantOutMin=[]  FilterDenConstantOutMax=[]  PCopyOutDataTypeStr=Inherit: Inherit via back propagation  PCopyOutMin=[]  PCopyOutMax=[]  NCopyOutDataTypeStr=Inherit: Inherit via back propagation  NCopyOutMin=[]  NCopyOutMax=[]  IntegratorContinuousStateAttributes=''  IntegratorStateMustResolveToSignalObject=off  IntegratorRTWStateStorageClass=Auto  FilterContinuousStateAttributes=''  FilterStateMustResolveToSignalObject=off  FilterRTWStateStorageClass=Auto  ParallelPVariant=InternalParameters  IdealPVariant=Disabled  IVariant=InternalParameters  DVariant=Disabled  IntegratorVariant=Discrete  SatVariant=Enabled  AWVariant=DiscClampingParallel  PCopyVariant=Disabled  TRVariant=Disabled  FdbkBlocksVariant=Forward  IdealPFdbkVariant=Disabled  SatFdbkVariant=Disabled  DerivativeFilterVariant=Disabled  NVariant=Disabled  NCopyVariant=Disabled_SignalSpec  FilterICVariant=Disabled  IntegratorICVariant=InternalICs  ExternalResetVariant=Disabled  TRSumVariant=Passthrough  SumFdbkVariant=Disabled  SumVariant=Sum_PI  TsampFilterVariant=InternalTs  TsampNgainVariant=Passthrough  TsampIntegralVariant=Disabled_SignalSpec  ExternalSaturationOutDataTypeStr=Inherit: Same as second input  DerivativeSourceVariant=Disabled  PreIntVariant=InternalPreInt
  Saturation : Saturate  UpperLimit=U_max_val  LowerLimit=-U_max_val
  Scope : Scope  NumInputPorts=4
      settings: ActiveDisplayYMinimum=2.7304984706864341  ActiveDisplayYMaximum=3.2653968597086265
  Step : Step  Commented=on  SampleTime=0
  Step1 : Step  Commented=on  SampleTime=0
  phi_ref_filtered : Outport
  u : Outport  Port=2
  wires:
  phi_ref/1 -> [phi_ref]
  phi_2_measured/1 -> [phi_2_measured]
  [phi_ref_filtered] -> phi_ref_filtered/1
  [u] -> u/1
  [phi_1_measured] -> Derivative/1
  Derivative/1 -> [dphi_1]
  [phi_2_measured] -> Derivative1/1
  Derivative1/1 -> [dphi_2]
  phi_1_measured/1 -> [phi_1_measured]
  i/1 -> [i]
  Minus/1 -> PID Controller/1
  [i_ref] -> Minus/1
  [i] -> Minus/2
  Minus2/1 -> PID Controller/3
  Minus1/1 -> PID Controller/2
  Constant1/1 -> Minus2/1
  Constant/1 -> Minus1/1
  [dphi_1] -> Gain/1
  Gain/1 -> [u_ff]
  [u_ff] -> Minus1/2
  [u_ff] -> Minus2/2
  PID Controller/1 -> [u_fb]
  [u_ff] -> Add/1
  [u_fb] -> Add/2
  Add/1 -> Saturation/1
  Saturation/1 -> [u]
  [i_ref] -> Mux/1
  [i] -> Mux/2
  Mux/1 -> Scope/3
  [u] -> Scope/4
  Step/1 -> Goto9/1
  Step1/1 -> Goto10/1
  Minus3/1 -> PID Controller1/1
  From16/1 -> Minus3/1
  From13/1 -> Minus3/2
  PID Controller1/1 -> Gain1/1
  [dphi_1_ref] -> Mux1/1
  [dphi_1] -> Mux1/2
  Mux1/1 -> Scope/2
  [dphi_2] -> Mux1/3
  Gain1/1 -> Goto11/1
  Minus4/1 -> PID Controller2/1
  PID Controller2/1 -> [i_ref_fb]
  [dphi_1_ref] -> Minus4/1
  [dphi_1] -> Minus4/2
  Minus5/1 -> PID Controller2/2
  Constant2/1 -> Minus5/1
  Minus6/1 -> PID Controller2/3
  Constant3/1 -> Minus6/1
  Gain3/1 -> [i_ref_ff]
  [i_ref_ff] -> Minus5/2
  [i_ref_ff] -> Minus6/2
  [phi_1_measured] -> Minus7/1
  [phi_2_measured] -> Minus7/2
  [i_ref_fb] -> Add1/1
  [i_ref_ff] -> Add1/2
  Add1/1 -> Gain4/1
  Gain4/1 -> [i_ref]
  Minus7/1 -> Gain2/1
  Gain2/1 -> Gain3/1
  Gain7/1 -> Goto17/1
  From29/1 -> Minus9/2
  From33/1 -> Add2/1
  From34/1 -> Add2/2
  Constant5/1 -> Minus10/1
  From30/1 -> Minus10/2
  From27/1 -> Minus8/2
  From28/1 -> Minus8/1
  PID Controller3/1 -> Goto15/1
  Minus10/1 -> PID Controller3/3
  Minus11/1 -> Gain6/1
  Minus9/1 -> PID Controller3/2
  Constant4/1 -> Minus9/1
  Add2/1 -> Gain7/1
  Gain6/1 -> Goto16/1
  Minus8/1 -> PID Controller3/1
  From31/1 -> Minus11/1
  From32/1 -> Minus11/2
  From40/1 -> Minus13/2
  From39/1 -> Minus13/1
  Minus13/1 -> Gain5/1
  Minus14/1 -> PID Controller4/1
  Minus15/1 -> PID Controller4/2
  Constant6/1 -> Minus15/1
  Gain5/1 -> Goto19/1
  Add3/1 -> Gain8/1
  PID Controller4/1 -> Goto18/1
  From38/1 -> Minus12/2
  From36/1 -> Minus14/1
  Constant7/1 -> Minus12/1
  From35/1 -> Minus14/2
  From37/1 -> Minus15/2
  From42/1 -> Add3/2
  From41/1 -> Add3/1
  Gain8/1 -> Goto20/1
  Minus12/1 -> PID Controller4/3
  Gain9/1 -> Goto21/1
  From44/1 -> Minus16/2
  Minus16/1 -> Gain9/1
  From45/1 -> Minus16/1
  From43/1 -> Add4/1
  From46/1 -> Add4/2
  Add4/1 -> Goto22/1
  PID Controller5/1 -> [dphi_1_ref]
  Minus17/1 -> PID Controller5/1
  [phi_2_measured] -> Minus17/2
  [phi_2_measured] -> Mux2/2
  [phi_ref] -> Mux2/1
  Mux2/1 -> Scope/1
  [phi_ref] -> Minus17/1

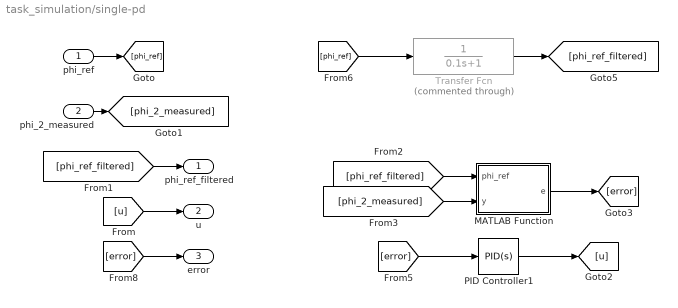
== system task_simulation/single-pd ==
  phi_ref : Inport
  phi_2_measured : Inport  Port=2
  MATLAB Function : MATLAB Function  TreatAsAtomicUnit=on
  PID Controller1 : slpidlib/PID Controller  Controller=PID  Form=Parallel  TimeDomain=Continuous-time  UseExternalTs=off  SampleTime=-1  IntegratorMethod=Forward Euler  FilterMethod=Forward Euler  ControllerParametersSource=internal  P=0.04  I=0  UseKiTs=off  D=0.04 * 0.0015  UseExternalDerivativeSource=off  N=1000  UseFilter=on  TunerSelectOption=Transfer Function Based (PID Tuner App)  InitialConditionSource=internal  InitialConditionForIntegrator=0  InitialConditionForFilter=0  DifferentiatorICPrevScaledInput=0  ExternalReset=none  TrackingMode=off  Kt=1  LimitOutput=on  SatLimitsSource=internal  UpperSaturationLimit=U_max_val  LowerSaturationLimit=-U_max_val  LinearizeAsGain=on  AntiWindupMode=clamping  Kb=1  LimitIntegrator=off  UpperIntegratorSaturationLimit=inf  LowerIntegratorSaturationLimit=-inf  POutMin=[]  POutMax=[]  IOutMin=[]  IOutMax=[]  DOutMin=[]  DOutMax=[]  NOutMin=[]  NOutMax=[]  SumOutMin=[]  SumOutMax=[]  SaturationOutMin=[]  SaturationOutMax=[]  PParamMin=[]  PParamMax=[]  IParamMin=[]  IParamMax=[]  DParamMin=[]  DParamMax=[]  NParamMin=[]  NParamMax=[]  KbParamMin=[]  KbParamMax=[]  KtParamMin=[]  KtParamMax=[]  KbOutMin=[]  KbOutMax=[]  KtOutMin=[]  KtOutMax=[]  IntegratorOutMin=[]  IntegratorOutMax=[]  FilterOutMin=[]  FilterOutMax=[]  SumI1OutMin=[]  SumI1OutMax=[]  SumI2OutMin=[]  SumI2OutMax=[]  SumI3OutMin=[]  SumI3OutMax=[]  SumI4OutMin=[]  SumI4OutMax=[]  SumDOutMin=[]  SumDOutMax=[]  DifferentiatorOutMin=[]  DifferentiatorOutMax=[]  FilterDiffOutCoefMin=[]  FilterDiffOutCoefMax=[]  ReciprocalOutMin=[]  ReciprocalOutMax=[]  SumDenOutMin=[]  SumDenOutMax=[]  SumNumOutMin=[]  SumNumOutMax=[]  DivideOutMin=[]  DivideOutMax=[]  UdiffTsProdOutMin=[]  UdiffTsProdOutMax=[]  NTsProdOutMin=[]  NTsProdOutMax=[]  UintegralTsProdOutMin=[]  UintegralTsProdOutMax=[]  UngainTsProdOutMin=[]  UngainTsProdOutMax=[]  ClampingZeroOutDataTypeStr=Inherit: Inherit via back propagation  ClampingZeroOutMin=[]  ClampingZeroOutMax=[]  FilterDenConstantOutDataTypeStr=Inherit: Inherit via back propagation  FilterDenConstantOutMin=[]  FilterDenConstantOutMax=[]  PCopyOutDataTypeStr=Inherit: Inherit via back propagation  PCopyOutMin=[]  PCopyOutMax=[]  NCopyOutDataTypeStr=Inherit: Inherit via back propagation  NCopyOutMin=[]  NCopyOutMax=[]  IntegratorContinuousStateAttributes=''  IntegratorStateMustResolveToSignalObject=off  IntegratorRTWStateStorageClass=Auto  FilterContinuousStateAttributes=''  FilterStateMustResolveToSignalObject=off  FilterRTWStateStorageClass=Auto  ParallelPVariant=InternalParameters  IdealPVariant=Disabled  IVariant=InternalParameters  DVariant=InternalParameters  IntegratorVariant=Continuous  SatVariant=Enabled  AWVariant=ContClampingParallel  PCopyVariant=Disabled  TRVariant=Disabled  FdbkBlocksVariant=Forward  IdealPFdbkVariant=Disabled  SatFdbkVariant=Disabled  DerivativeFilterVariant=ContFilter  NVariant=InternalParameters  NCopyVariant=Disabled  FilterICVariant=InternalICsFilter  IntegratorICVariant=InternalICs  ExternalResetVariant=Disabled  TRSumVariant=Passthrough  SumFdbkVariant=Disabled  SumVariant=Sum_PID  TsampFilterVariant=InternalTs  TsampNgainVariant=Passthrough  TsampIntegralVariant=Disabled_SignalSpec  ExternalSaturationOutDataTypeStr=Inherit: Same as second input  DerivativeSourceVariant=ErrorSignal  PreIntVariant=InternalPreInt
  Transfer Fcn : TransferFcn  Commented=through  Denominator=[0.1 1]
  phi_ref_filtered : Outport
  u : Outport  Port=2
  error : Outport  Port=3
  wires:
  MATLAB Function/1(e) -> [error]
  Transfer Fcn/1 -> [phi_ref_filtered]
  [phi_2_measured] -> MATLAB Function/2(y)
  [phi_ref] -> Transfer Fcn/1
  [phi_ref_filtered] -> MATLAB Function/1(phi_ref)
  phi_ref/1 -> [phi_ref]
  phi_2_measured/1 -> [phi_2_measured]
  [phi_ref_filtered] -> phi_ref_filtered/1
  [u] -> u/1
  PID Controller1/1 -> [u]
  [error] -> PID Controller1/1
  [error] -> error/1

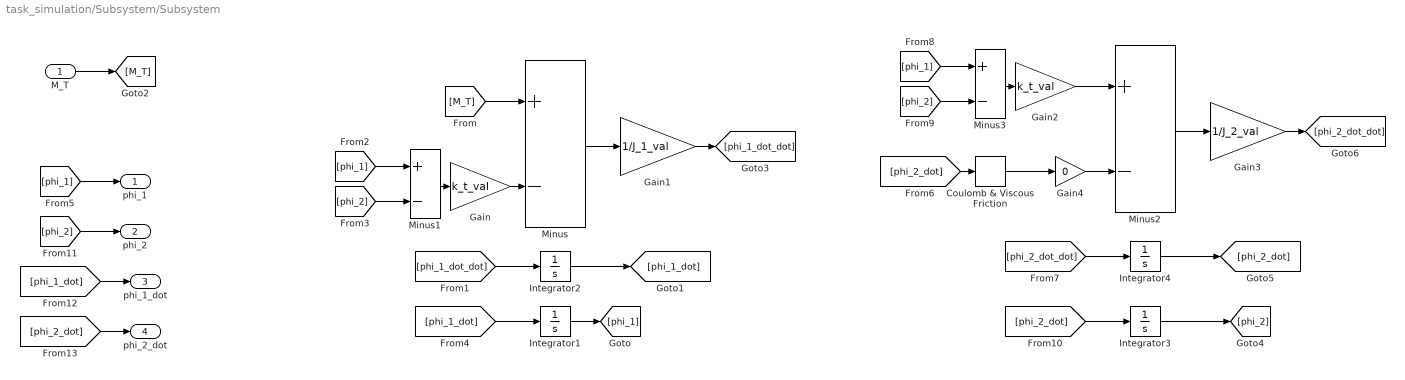
== system task_simulation/Subsystem/Subsystem ==
  M_T : Inport
  Coulomb & Viscous Friction : simulink/Discontinuities/Coulomb & Viscous Friction  offset=0.5  gain=0
  Gain : Gain  Gain=k_t_val
  Gain1 : Gain  Gain=1/J_1_val
  Gain2 : Gain  Gain=k_t_val
  Gain3 : Gain  Gain=1/J_2_val
  Gain4 : Gain  Gain=0
  Integrator{1..4} (4 alike) : Integrator
  Minus{,1..3} (4 alike) : Sum  Inputs=+-
  phi_1 : Outport
  phi_2 : Outport  Port=2
  phi_1_dot : Outport  Port=3
  phi_2_dot : Outport  Port=4
  wires:
  [phi_1_dot] -> Integrator1/1
  Integrator1/1 -> [phi_1]
  Integrator2/1 -> [phi_1_dot]
  [phi_1_dot_dot] -> Integrator2/1
  M_T/1 -> [M_T]
  [M_T] -> Minus/1
  Minus1/1 -> Gain/1
  [phi_1] -> Minus1/1
  [phi_2] -> Minus1/2
  Gain/1 -> Minus/2
  Minus/1 -> Gain1/1
  Gain1/1 -> [phi_1_dot_dot]
  [phi_1] -> phi_1/1
  [phi_2_dot] -> Integrator3/1
  Integrator3/1 -> [phi_2]
  [phi_2_dot_dot] -> Integrator4/1
  Minus2/1 -> Gain3/1
  [phi_2] -> Minus3/2
  Integrator4/1 -> [phi_2_dot]
  Minus3/1 -> Gain2/1
  Gain3/1 -> [phi_2_dot_dot]
  [phi_1] -> Minus3/1
  Gain2/1 -> Minus2/1
  Coulomb & Viscous Friction/1 -> Gain4/1
  [phi_2] -> phi_2/1
  [phi_1_dot] -> phi_1_dot/1
  [phi_2_dot] -> phi_2_dot/1
  [phi_2_dot] -> Coulomb & Viscous Friction/1
  Gain4/1 -> Minus2/2

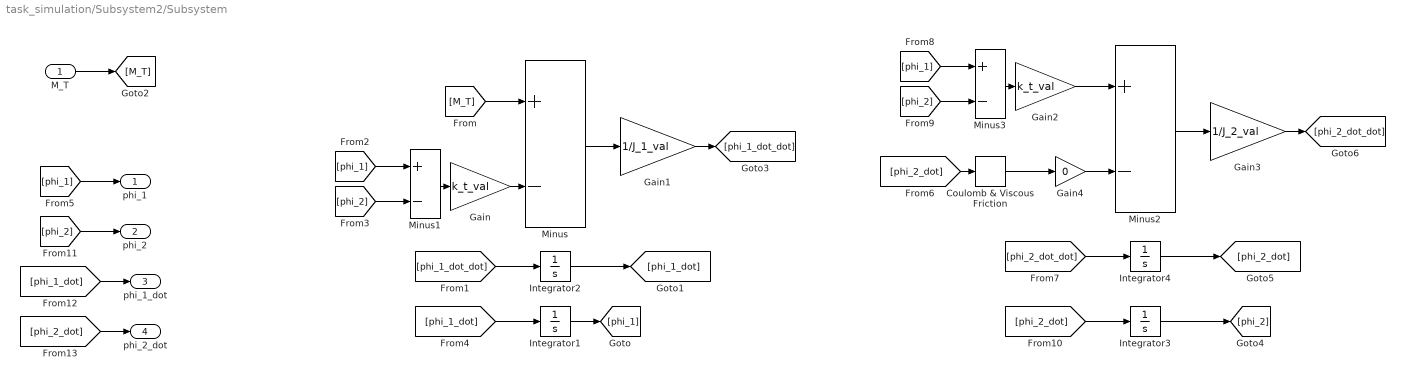
== system task_simulation/Subsystem2/Subsystem ==
  M_T : Inport
  Coulomb & Viscous Friction : simulink/Discontinuities/Coulomb & Viscous Friction  offset=0.5  gain=0
  Gain : Gain  Gain=k_t_val
  Gain1 : Gain  Gain=1/J_1_val
  Gain2 : Gain  Gain=k_t_val
  Gain3 : Gain  Gain=1/J_2_val
  Gain4 : Gain  Gain=0
  Integrator{1..4} (4 alike) : Integrator
  Minus{,1..3} (4 alike) : Sum  Inputs=+-
  phi_1 : Outport
  phi_2 : Outport  Port=2
  phi_1_dot : Outport  Port=3
  phi_2_dot : Outport  Port=4
  wires:
  [phi_1_dot] -> Integrator1/1
  Integrator1/1 -> [phi_1]
  Integrator2/1 -> [phi_1_dot]
  [phi_1_dot_dot] -> Integrator2/1
  M_T/1 -> [M_T]
  [M_T] -> Minus/1
  Minus1/1 -> Gain/1
  [phi_1] -> Minus1/1
  [phi_2] -> Minus1/2
  Gain/1 -> Minus/2
  Minus/1 -> Gain1/1
  Gain1/1 -> [phi_1_dot_dot]
  [phi_1] -> phi_1/1
  [phi_2_dot] -> Integrator3/1
  Integrator3/1 -> [phi_2]
  [phi_2_dot_dot] -> Integrator4/1
  Minus2/1 -> Gain3/1
  [phi_2] -> Minus3/2
  Integrator4/1 -> [phi_2_dot]
  Minus3/1 -> Gain2/1
  Gain3/1 -> [phi_2_dot_dot]
  [phi_1] -> Minus3/1
  Gain2/1 -> Minus2/1
  Coulomb & Viscous Friction/1 -> Gain4/1
  [phi_2] -> phi_2/1
  [phi_1_dot] -> phi_1_dot/1
  [phi_2_dot] -> phi_2_dot/1
  [phi_2_dot] -> Coulomb & Viscous Friction/1
  Gain4/1 -> Minus2/2

== matlab function task_simulation/single-pd/MATLAB Function ==
  data: phi_ref input; e output; y input
function e = angle_error(phi_ref, y)
    delta = phi_ref - y;
    e = atan2d(sind(delta), cosd(delta));
end
